simulink model "Atuadores"  (R2020a)
settings: Solver=VariableStepAuto  StartTime=0.0  StopTime=10.0  RelTol=1e-3
values from neighbouring files (symbols this model uses):
  A_vec = [0.01; 0.01; 0.01]    [Variaveis_Atuadores.m]
  A_wire_mt = ((10e-3)^2)*pi    (= 0.000314159265359)    [Variaveis_Atuadores.m]
  alpha_0_mt = 3.9e-3    (= 0.0039)    [Variaveis_Atuadores.m]
  Ctrl_PWM = [1; 1; 1]    [Variaveis_Atuadores.m]
  K_x = 1e-4    (= 0.0001)    [Variaveis_Atuadores.m]
  K_y = 1e-4    (= 0.0001)    [Variaveis_Atuadores.m]
  K_z = 1e-4    (= 0.0001)    [Variaveis_Atuadores.m]
  Mag_I = 1e-9 * [21038.82; -2074.02; 17521.53]    [Variaveis_Atuadores.m]    (also in Variaveis_Sensores.m = 1e-9 * [-16039.3481; 5746.0765; 32029.4825])
  n_mt = 200    [Variaveis_Atuadores.m]
  p_wire = (10e-3)*2*pi    (= 0.0628318530718)    [Variaveis_Atuadores.m]
  sigma_0_mt = 1.72e-8    (= 1.72e-08)    [Variaveis_Atuadores.m]
  T_0_mt = 293    [Variaveis_Atuadores.m]
  v_I_S = [-15.5; -85.5; -85.5]    [Variaveis_Atuadores.m]    (also in Variaveis_Sensores.m)
libraries: sharedutil x3, aerolibutil x1, sharedtransform x1
settings Model: Creator=kakat  LastModifiedBy=kakat

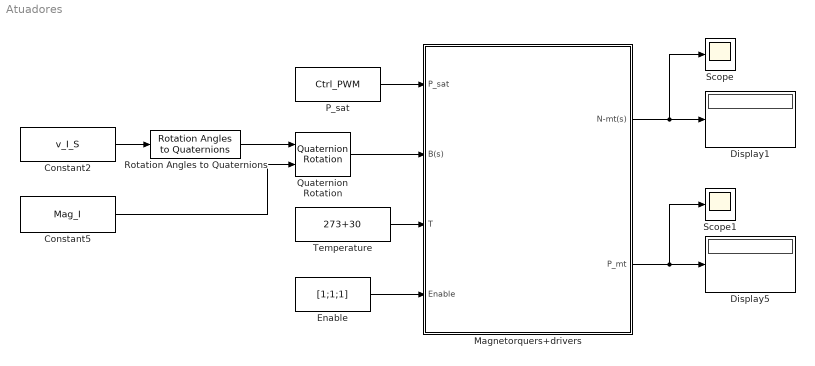
== system Atuadores ==
  Constant2 : Constant  Value=v_I_S
  Constant5 : Constant  Value=Mag_I
  Display1 : Display
  Display5 : Display
  Enable : Constant  Value=[1;1;1]
  Magnetorquers+drivers : Subsystem
  P_sat : Constant  Value=Ctrl_PWM
  Quaternion Rotation : aerolibutil/Quaternion Rotation
  Rotation Angles to Quaternions : sharedtransform/Rotation Angles to Quaternions  rotationOrder=ZYX  aMode=aMode
      settings: SourceProductBaseCode=AE,PW,MT,VE,VP
  Scope : Scope
  Scope1 : Scope
  Temperature : Constant  Value=273+30
  wires:
  Temperature/1 -> Magnetorquers+drivers/3(T)
  P_sat/1 -> Magnetorquers+drivers/1(P_sat)
  Enable/1 -> Magnetorquers+drivers/4(Enable)
  Magnetorquers+drivers/2(P_mt) -> Scope1/1, Display5/1
  Magnetorquers+drivers/1(N-mt(s)) -> Display1/1, Scope/1
  Rotation Angles to Quaternions/1 -> Quaternion Rotation/1
  Constant2/1 -> Rotation Angles to Quaternions/1
  Constant5/1 -> Quaternion Rotation/2
  Quaternion Rotation/1 -> Magnetorquers+drivers/2(B(s))

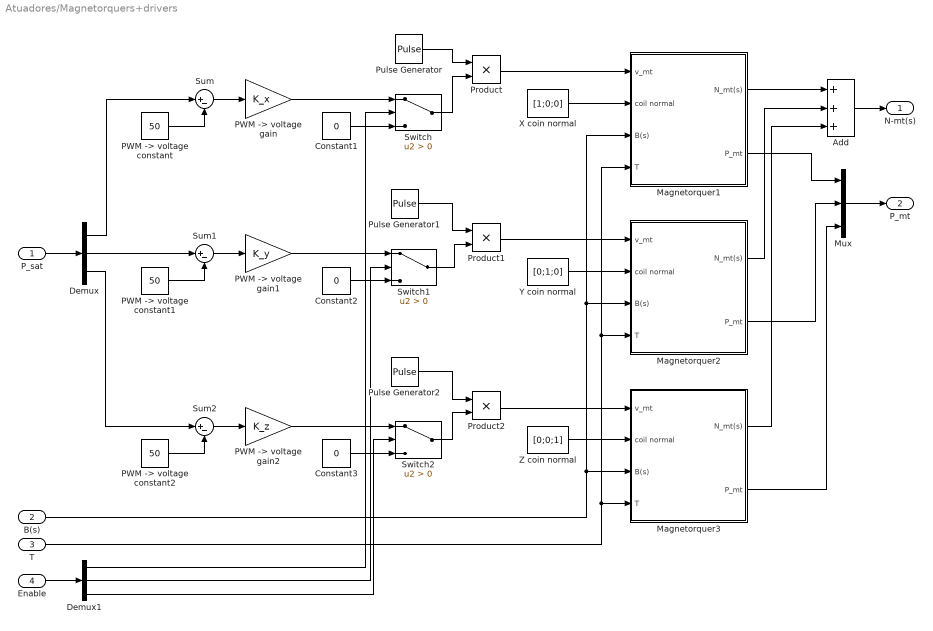
== system Atuadores/Magnetorquers+drivers ==
  P_sat : Inport
  B(s) : Inport  Port=2
  T : Inport  Port=3
  Enable : Inport  Port=4
  Add : Sum  Inputs=+++
  Constant1 : Constant  Value=0
  Constant2 : Constant  Value=0
  Constant3 : Constant  Value=0
  Demux : Demux  Outputs=3
  Demux1 : Demux  Outputs=3
  Magnetorquer1 : Subsystem
  Magnetorquer2 : Subsystem
  Magnetorquer3 : Subsystem
  Mux : Mux  Inputs=3
  "PWM -> voltage constant" : Constant  Value=50
  "PWM -> voltage constant1" : Constant  Value=50
  "PWM -> voltage constant2" : Constant  Value=50
  "PWM -> voltage gain" : Gain  Gain=K_x
  "PWM -> voltage gain1" : Gain  Gain=K_y
  "PWM -> voltage gain2" : Gain  Gain=K_z
  Product : Product
  Product1 : Product
  Product2 : Product
  Pulse Generator : DiscretePulseGenerator  PulseType=Time based  Period=0.1  PulseWidth=50
  Pulse Generator1 : DiscretePulseGenerator  PulseType=Time based  Period=0.1  PulseWidth=50
  Pulse Generator2 : DiscretePulseGenerator  PulseType=Time based  Period=0.1  PulseWidth=50
  Sum : Sum  Inputs=|+-
  Sum1 : Sum  Inputs=|+-
  Sum2 : Sum  Inputs=|+-
  Switch : Switch  Criteria=u2 > Threshold
  Switch1 : Switch  Criteria=u2 > Threshold
  Switch2 : Switch  Criteria=u2 > Threshold
  X coin normal : Constant  Value=[1;0;0]
  Y coin normal : Constant  Value=[0;1;0]
  Z coin normal : Constant  Value=[0;0;1]
  N-mt(s) : Outport
  P_mt : Outport  Port=2
  wires:
  Sum/1 -> "PWM -> voltage gain"/1
  Constant1/1 -> Switch/3
  Pulse Generator/1 -> Product/1
  Switch/1 -> Product/2
  "PWM -> voltage gain"/1 -> Switch/1
  Product/1 -> Magnetorquer1/1(v_mt)
  Enable/1 -> Demux1/1
  P_sat/1 -> Demux/1
  "PWM -> voltage constant"/1 -> Sum/2
  Demux1/1 -> Switch/2
  Demux/3 -> Sum2/1
  X coin normal/1 -> Magnetorquer1/2(coil normal)
  B(s)/1 -> Magnetorquer1/3(B(s)), Magnetorquer2/3(B(s)), Magnetorquer3/3(B(s))
  T/1 -> Magnetorquer3/4(T), Magnetorquer1/4(T), Magnetorquer2/4(T)
  Mux/1 -> P_mt/1
  Y coin normal/1 -> Magnetorquer2/2(coil normal)
  Product1/1 -> Magnetorquer2/1(v_mt)
  Pulse Generator1/1 -> Product1/1
  "PWM -> voltage gain1"/1 -> Switch1/1
  Sum1/1 -> "PWM -> voltage gain1"/1
  "PWM -> voltage constant1"/1 -> Sum1/2
  Switch1/1 -> Product1/2
  Constant2/1 -> Switch1/3
  Z coin normal/1 -> Magnetorquer3/2(coil normal)
  Product2/1 -> Magnetorquer3/1(v_mt)
  Pulse Generator2/1 -> Product2/1
  "PWM -> voltage gain2"/1 -> Switch2/1
  Sum2/1 -> "PWM -> voltage gain2"/1
  "PWM -> voltage constant2"/1 -> Sum2/2
  Switch2/1 -> Product2/2
  Constant3/1 -> Switch2/3
  Demux/2 -> Sum1/1
  Demux1/2 -> Switch1/2
  Demux1/3 -> Switch2/2
  Demux/1 -> Sum/1
  Magnetorquer1/1(N_mt(s)) -> Add/1
  Magnetorquer2/1(N_mt(s)) -> Add/2
  Magnetorquer3/1(N_mt(s)) -> Add/3
  Magnetorquer1/2(P_mt) -> Mux/1
  Magnetorquer2/2(P_mt) -> Mux/2
  Magnetorquer3/2(P_mt) -> Mux/3
  Add/1 -> N-mt(s)/1

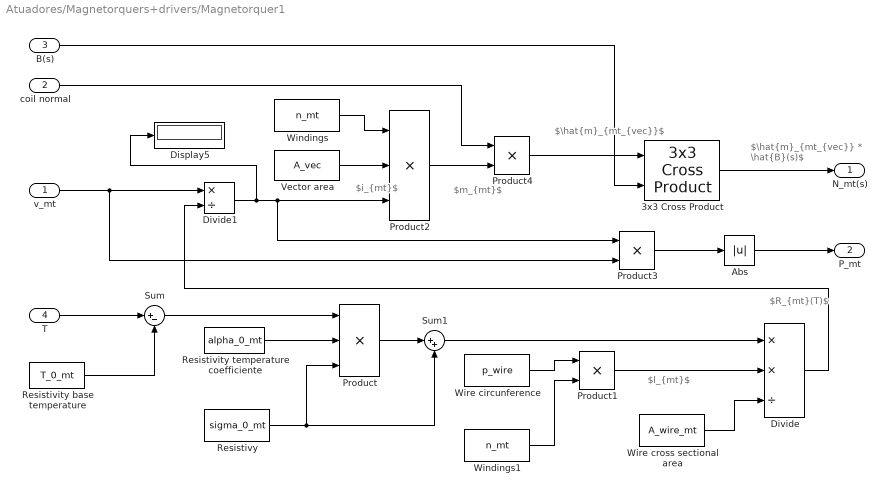
== system Atuadores/Magnetorquers+drivers/Magnetorquer1 ==
  note: $l_{mt}$
  note: $\hat{m}_{mt_{vec}} * \hat{B}(s)$
  note: $\hat{m}_{mt_{vec}}$
  note: $m_{mt}$
  note: $i_{mt}$
  note: $R_{mt}(T)$
  v_mt : Inport
  coil normal : Inport  Port=2
  B(s) : Inport  Port=3
  T : Inport  Port=4
  3x3 Cross Product : sharedutil/3x3 Cross Product  aMode=aMode
      settings: SourceProductBaseCode=AE,PW,MT,VE,VP
  Abs : Abs
  Display5 : Display
  Divide : Product  Inputs=**/
  Divide1 : Product  Inputs=*/
  Product : Product  Inputs=3
  Product1 : Product
  Product2 : Product  Inputs=3
  Product3 : Product
  Product4 : Product
  Resistivity temperature coefficiente : Constant  Value=alpha_0_mt
  Resistivity base temperature : Constant  Value=T_0_mt
  Resistivy : Constant  Value=sigma_0_mt
  Sum : Sum  Inputs=|+-
  Sum1 : Sum  Inputs=|++
  Vector area : Constant  Value=A_vec
  Windings : Constant  Value=n_mt
  Windings1 : Constant  Value=n_mt
  Wire circunference : Constant  Value=p_wire
  Wire cross sectional area : Constant  Value=A_wire_mt
  N_mt(s) : Outport
  P_mt : Outport  Port=2
  wires:
  Sum/1 -> Product/1
  T/1 -> Sum/1
  Resistivity temperature coefficiente/1 -> Product/2
  Product/1 -> Sum1/1
  Resistivity base temperature/1 -> Sum/2
  Windings1/1 -> Product1/2
  v_mt/1 -> Divide1/1, Product3/2
  Divide/1 -> Divide1/2
  Divide1/1 -> Display5/1, Product3/1, Product2/3
  Windings/1 -> Product2/1
  Vector area/1 -> Product2/2
  Abs/1 -> P_mt/1
  Product3/1 -> Abs/1
  Product2/1 -> Product4/2
  coil normal/1 -> Product4/1
  Product4/1 -> 3x3 Cross Product/1
  B(s)/1 -> 3x3 Cross Product/2
  3x3 Cross Product/1 -> N_mt(s)/1
  Wire circunference/1 -> Product1/1
  Wire cross sectional area/1 -> Divide/3
  Product1/1 -> Divide/2
  Resistivy/1 -> Sum1/2, Product/3
  Sum1/1 -> Divide/1

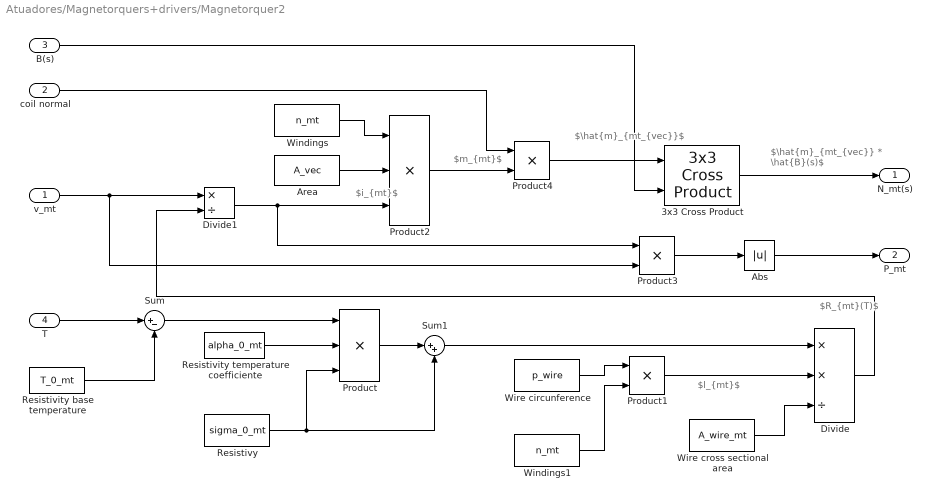
== system Atuadores/Magnetorquers+drivers/Magnetorquer2 ==
  note: $l_{mt}$
  note: $\hat{m}_{mt_{vec}} * \hat{B}(s)$
  note: $\hat{m}_{mt_{vec}}$
  note: $m_{mt}$
  note: $i_{mt}$
  note: $R_{mt}(T)$
  v_mt : Inport
  coil normal : Inport  Port=2
  B(s) : Inport  Port=3
  T : Inport  Port=4
  3x3 Cross Product : sharedutil/3x3 Cross Product  aMode=aMode
      settings: SourceProductBaseCode=AE,PW,MT,VE,VP
  Abs : Abs
  Area : Constant  Value=A_vec
  Divide : Product  Inputs=**/
  Divide1 : Product  Inputs=*/
  Product : Product  Inputs=3
  Product1 : Product
  Product2 : Product  Inputs=3
  Product3 : Product
  Product4 : Product
  Resistivity temperature coefficiente : Constant  Value=alpha_0_mt
  Resistivity base temperature : Constant  Value=T_0_mt
  Resistivy : Constant  Value=sigma_0_mt
  Sum : Sum  Inputs=|+-
  Sum1 : Sum  Inputs=|++
  Windings : Constant  Value=n_mt
  Windings1 : Constant  Value=n_mt
  Wire circunference : Constant  Value=p_wire
  Wire cross sectional area : Constant  Value=A_wire_mt
  N_mt(s) : Outport
  P_mt : Outport  Port=2
  wires:
  Sum/1 -> Product/1
  T/1 -> Sum/1
  Resistivity temperature coefficiente/1 -> Product/2
  Product/1 -> Sum1/1
  Resistivity base temperature/1 -> Sum/2
  Windings1/1 -> Product1/2
  v_mt/1 -> Divide1/1, Product3/2
  Divide/1 -> Divide1/2
  Divide1/1 -> Product3/1, Product2/3
  Windings/1 -> Product2/1
  Area/1 -> Product2/2
  Abs/1 -> P_mt/1
  Product3/1 -> Abs/1
  Product2/1 -> Product4/2
  coil normal/1 -> Product4/1
  Product4/1 -> 3x3 Cross Product/1
  B(s)/1 -> 3x3 Cross Product/2
  3x3 Cross Product/1 -> N_mt(s)/1
  Wire circunference/1 -> Product1/1
  Wire cross sectional area/1 -> Divide/3
  Product1/1 -> Divide/2
  Resistivy/1 -> Sum1/2, Product/3
  Sum1/1 -> Divide/1

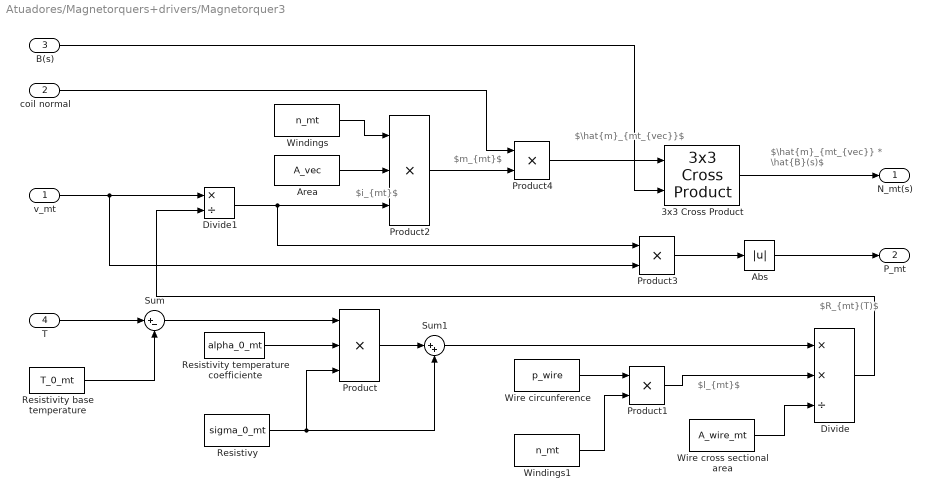
== system Atuadores/Magnetorquers+drivers/Magnetorquer3 ==
  note: $l_{mt}$
  note: $\hat{m}_{mt_{vec}} * \hat{B}(s)$
  note: $\hat{m}_{mt_{vec}}$
  note: $m_{mt}$
  note: $i_{mt}$
  note: $R_{mt}(T)$
  v_mt : Inport
  coil normal : Inport  Port=2
  B(s) : Inport  Port=3
  T : Inport  Port=4
  3x3 Cross Product : sharedutil/3x3 Cross Product  aMode=aMode
      settings: SourceProductBaseCode=AE,PW,MT,VE,VP
  Abs : Abs
  Area : Constant  Value=A_vec
  Divide : Product  Inputs=**/
  Divide1 : Product  Inputs=*/
  Product : Product  Inputs=3
  Product1 : Product
  Product2 : Product  Inputs=3
  Product3 : Product
  Product4 : Product
  Resistivity temperature coefficiente : Constant  Value=alpha_0_mt
  Resistivity base temperature : Constant  Value=T_0_mt
  Resistivy : Constant  Value=sigma_0_mt
  Sum : Sum  Inputs=|+-
  Sum1 : Sum  Inputs=|++
  Windings : Constant  Value=n_mt
  Windings1 : Constant  Value=n_mt
  Wire circunference : Constant  Value=p_wire
  Wire cross sectional area : Constant  Value=A_wire_mt
  N_mt(s) : Outport
  P_mt : Outport  Port=2
  wires:
  Sum/1 -> Product/1
  T/1 -> Sum/1
  Resistivity temperature coefficiente/1 -> Product/2
  Product/1 -> Sum1/1
  Resistivity base temperature/1 -> Sum/2
  Windings1/1 -> Product1/2
  v_mt/1 -> Divide1/1, Product3/2
  Divide/1 -> Divide1/2
  Divide1/1 -> Product3/1, Product2/3
  Windings/1 -> Product2/1
  Area/1 -> Product2/2
  Abs/1 -> P_mt/1
  Product3/1 -> Abs/1
  Product2/1 -> Product4/2
  coil normal/1 -> Product4/1
  Product4/1 -> 3x3 Cross Product/1
  B(s)/1 -> 3x3 Cross Product/2
  3x3 Cross Product/1 -> N_mt(s)/1
  Wire circunference/1 -> Product1/1
  Wire cross sectional area/1 -> Divide/3
  Product1/1 -> Divide/2
  Resistivy/1 -> Sum1/2, Product/3
  Sum1/1 -> Divide/1
